simulink model "undirect_graph_consensus"  (R2020a)
settings: Solver=FixedStepAuto  StartTime=0.0  StopTime=10.0  FixedStep=0.0001  RelTol=1e-3
libraries: fod x1
settings Model: Creator=WangQipeng  LastModifiedBy=WangQipeng

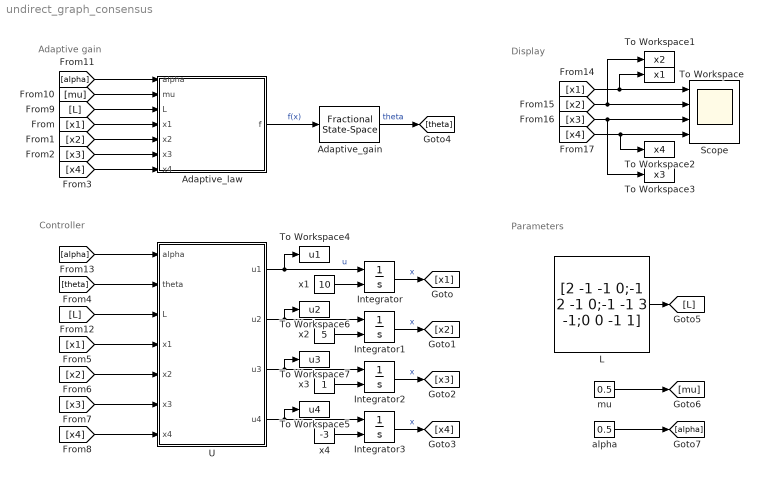
== system undirect_graph_consensus ==
  note: Controller
  note: Adaptive gain
  note: Display
  note: Parameters
  Adaptive_gain : fod/Fractional State-Space  A=0  B=1  C=1  D=0  q=0.5  iniOff=[0]  freqRange=[0.0001 10000]  approxNum=5  useRef=off  mask(FOSS){}
      settings: SourceProductName=FOMCON Toolbox
      mask Display: disp(['D^\beta \theta=f(x)'], 'TeXMode', 'On');
  Adaptive_law : MATLAB Function  TreatAsAtomicUnit=on
  Integrator{,1..3} (4 alike) : Integrator  InitialConditionSource=external  InitialCondition=1
  L : Constant  Value=[2 -1 -1 0;-1 2 -1 0;-1 -1 3 -1;0 0 -1 1]
  Scope : Scope  NumInputPorts=4
  To Workspace : ToWorkspace  VariableName=x1  SaveFormat=Timeseries  SampleTime=-1
  To Workspace1 : ToWorkspace  VariableName=x2  SaveFormat=Timeseries  SampleTime=-1
  To Workspace2 : ToWorkspace  VariableName=x4  SaveFormat=Timeseries  SampleTime=-1
  To Workspace3 : ToWorkspace  VariableName=x3  SaveFormat=Timeseries  SampleTime=-1
  To Workspace4 : ToWorkspace  VariableName=u1  SaveFormat=Timeseries  SampleTime=-1
  To Workspace5 : ToWorkspace  VariableName=u4  SaveFormat=Timeseries  SampleTime=-1
  To Workspace6 : ToWorkspace  VariableName=u2  SaveFormat=Timeseries  SampleTime=-1
  To Workspace7 : ToWorkspace  VariableName=u3  SaveFormat=Timeseries  SampleTime=-1
  U : MATLAB Function  TreatAsAtomicUnit=on
  alpha : Constant  Value=0.5
  mu : Constant  Value=0.5
  x1 : Constant  Value=10
  x2 : Constant  Value=5
  x3 : Constant
  x4 : Constant  Value=-3
  wires:
  U/1(u1) -> To Workspace4/1, Integrator/1  "u"
  Adaptive_law/1(f) -> Adaptive_gain/1  "f(x)"
  U/2(u2) -> To Workspace6/1, Integrator1/1
  U/3(u3) -> To Workspace7/1, Integrator2/1
  U/4(u4) -> To Workspace5/1, Integrator3/1
  Integrator/1 -> [x1]  "x"
  [x1] -> Adaptive_law/4(x1)
  Integrator1/1 -> [x2]  "x"
  Integrator2/1 -> [x3]  "x"
  Integrator3/1 -> [x4]  "x"
  [x2] -> Adaptive_law/5(x2)
  [x3] -> Adaptive_law/6(x3)
  [x4] -> Adaptive_law/7(x4)
  Adaptive_gain/1 -> [theta]  "theta"
  [theta] -> U/2(theta)
  [x3] -> U/6(x3)
  [x4] -> U/7(x4)
  [x1] -> U/4(x1)
  [x2] -> U/5(x2)
  L/1 -> [L]
  [L] -> Adaptive_law/3(L)
  mu/1 -> [mu]
  alpha/1 -> [alpha]
  [mu] -> Adaptive_law/2(mu)
  [alpha] -> Adaptive_law/1(alpha)
  [L] -> U/3(L)
  [alpha] -> U/1(alpha)
  x1/1 -> Integrator/2
  x2/1 -> Integrator1/2
  x3/1 -> Integrator2/2
  x4/1 -> Integrator3/2
  [x1] -> To Workspace/1, Scope/1
  [x2] -> Scope/2, To Workspace1/1
  [x3] -> Scope/3, To Workspace3/1
  [x4] -> Scope/4, To Workspace2/1

== matlab function undirect_graph_consensus/U ==
  data: alpha input; u1 output; theta input; L input; x1 input; x2 input; x3 input; x4 input; u2 output; u3 output; u4 output
function [u1,u2,u3,u4] = protocol(alpha,theta,L,x1,x2,x3,x4)
x = [x1;x2;x3;x4];
temp = L * x;
temp_u1 = temp(1);
temp_u2 = temp(2);
temp_u3 = temp(3);
temp_u4 = temp(4);

u1 = -theta * sign(temp_u1) * abs(temp_u1)^(1-alpha);
u2 = -theta * sign(temp_u2) * abs(temp_u2)^(1-alpha);
u3 = -theta * sign(temp_u3) * abs(temp_u3)^(1-alpha);
u4 = -theta * sign(temp_u4) * abs(temp_u4)^(1-alpha);

== matlab function undirect_graph_consensus/Adaptive_law ==
  data: alpha input; f output; mu input; L input; x1 input; x2 input; x3 input; x4 input
function f = Lyapunov_Like(alpha,mu,L,x1,x2,x3,x4)
x = [x1;x2;x3;x4];
P_L = 2 * x' * L * x;
f = mu * abs(P_L)^(alpha/2);
